simulink model "TrajectoryTracking_2015b_00"  (R2017a)
settings: Solver=ode45  StartTime=0.0  StopTime=200  RelTol=1e-3
values from neighbouring files (symbols this model uses):
  B_input = B_T    [ErrorDynamicsControllerDesign.m]
  tau_d_1 = C_RB1+C_A1+D1+G1    [DesiredInputOptimalConfiguration.m]
  tau_d_2 = C_RB2+C_A2+D2+G2    [DesiredInputOptimalConfiguration.m]
  tau_d_3 = C_RB3+C_A3+D3+G3    [DesiredInputOptimalConfiguration.m]
  tau_d_4 = C_RB4+C_A4+D4+G4    [DesiredInputOptimalConfiguration.m]
  tau_d_5 = C_RB5+C_A5+D5+G5    [DesiredInputOptimalConfiguration.m]
  tau_d_6 = C_RB6+C_A6+D6+G6    [DesiredInputOptimalConfiguration.m]
  tau_d_7 = C_RB7+C_A7+D7+G7    [DesiredInputOptimalConfiguration.m]
undefined symbols (not defined in the file or in its folder): angular_velocity_pitch_1, angular_velocity_pitch_2, angular_velocity_pitch_3, angular_velocity_pitch_4, angular_velocity_pitch_5, angular_velocity_pitch_6, angular_velocity_roll_1, angular_velocity_roll_2, angular_velocity_roll_3, angular_velocity_roll_4, angular_velocity_roll_5, angular_velocity_roll_6, angular_velocity_roll_7, angular_velocity_yaw_1, angular_velocity_yaw_2, angular_velocity_yaw_3, angular_velocity_yaw_4, angular_velocity_yaw_5, angular_velocity_yaw_6, angular_velocity_yaw_7, K1, K2, K3, K4, K5, K6, K7, linear_velocity_x_1, linear_velocity_x_2, linear_velocity_x_3, linear_velocity_x_4, linear_velocity_x_5, linear_velocity_x_6, linear_velocity_x_7, linear_velocity_y_1, linear_velocity_y_2, linear_velocity_y_3, linear_velocity_y_4, linear_velocity_y_5, linear_velocity_y_6, linear_velocity_y_7, linear_velocity_z_1, linear_velocity_z_2, linear_velocity_z_3, linear_velocity_z_4, linear_velocity_z_5, linear_velocity_z_6, linear_velocity_z_7, pitch_angle_1, pitch_angle_2, pitch_angle_3, pitch_angle_4, pitch_angle_5, pitch_angle_6, pitch_angle_7, roll_angle_1, roll_angle_2, roll_angle_3, roll_angle_4, roll_angle_5 ... (+52)
undefined symbols (not defined in the file): b_T1_optimized, b_T2_optimized, b_T3_optimized, b_T4_optimized, b_T5_optimized, b_T6_optimized, d_T1_optimized, d_T2_optimized, d_T3_optimized, d_T4_optimized, d_T5_optimized, d_T6_optimized, r_T1_optimized, r_T2_optimized, r_T3_optimized, r_T4_optimized, r_T5_optimized, r_T6_optimized
libraries: sharedtransform x1, shared6dofsys x1
(part 2 of 2)

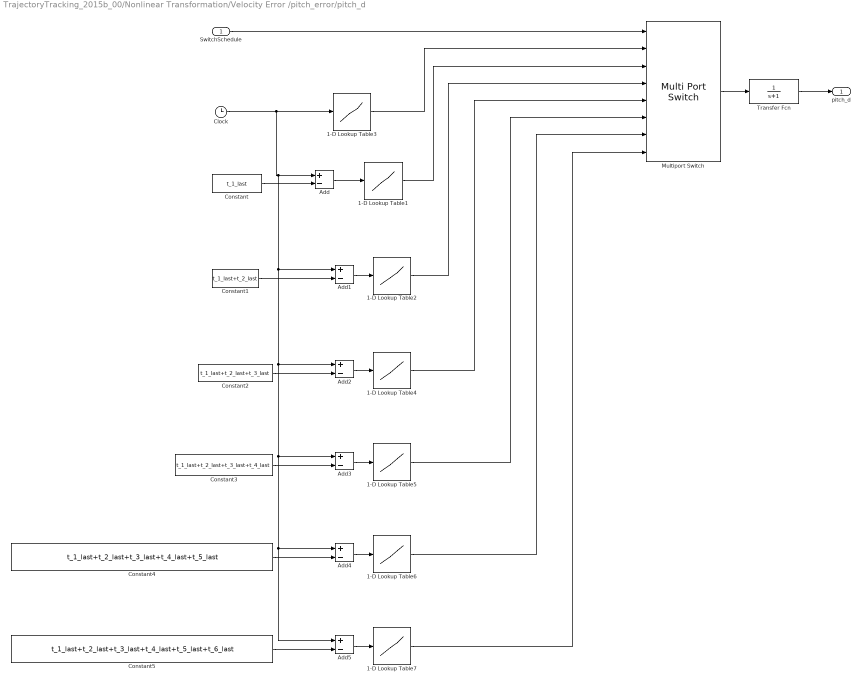
== system TrajectoryTracking_2015b_00/Nonlinear Transformation/Velocity Error /pitch_error/pitch_d ==
  SwitchSchedule : Inport
  1-D Lookup Table1 : Lookup_n-D  NumberOfTableDimensions=1  BreakpointsForDimension1=t_e_2  Table=angular_velocity_pitch_2  InternalRulePriority=Speed  RndMeth=Simplest  InputSameDT=on
  1-D Lookup Table2 : Lookup_n-D  NumberOfTableDimensions=1  BreakpointsForDimension1=t_e_3  Table=angular_velocity_pitch_3  InternalRulePriority=Speed  RndMeth=Simplest  InputSameDT=on
  1-D Lookup Table3 : Lookup_n-D  NumberOfTableDimensions=1  BreakpointsForDimension1=t_e_1  Table=angular_velocity_pitch_1  InternalRulePriority=Speed  RndMeth=Simplest  InputSameDT=on
  1-D Lookup Table4 : Lookup_n-D  NumberOfTableDimensions=1  BreakpointsForDimension1=t_e_4  Table=angular_velocity_pitch_4  InternalRulePriority=Speed  RndMeth=Simplest  InputSameDT=on
  1-D Lookup Table5 : Lookup_n-D  NumberOfTableDimensions=1  BreakpointsForDimension1=t_e_5  Table=angular_velocity_pitch_5  InternalRulePriority=Speed  RndMeth=Simplest  InputSameDT=on
  1-D Lookup Table6 : Lookup_n-D  NumberOfTableDimensions=1  BreakpointsForDimension1=t_e_6  Table=angular_velocity_pitch_6  InternalRulePriority=Speed  RndMeth=Simplest  InputSameDT=on
  1-D Lookup Table7 : Lookup_n-D  NumberOfTableDimensions=1  BreakpointsForDimension1=t_e_6  Table=angular_velocity_pitch_6  InternalRulePriority=Speed  RndMeth=Simplest  InputSameDT=on
  Add{,1..5} (6 alike) : Sum  Inputs=+-
  Clock : Clock
  Constant : Constant  Value=t_1_last
  Constant1 : Constant  Value=t_1_last+t_2_last
  Constant2 : Constant  Value=t_1_last+t_2_last+t_3_last
  Constant3 : Constant  Value=t_1_last+t_2_last+t_3_last+t_4_last
  Constant4 : Constant  Value=t_1_last+t_2_last+t_3_last+t_4_last+t_5_last
  Constant5 : Constant  Value=t_1_last+t_2_last+t_3_last+t_4_last+t_5_last+t_6_last
  Multiport Switch : MultiPortSwitch  Inputs=7
  Transfer Fcn : TransferFcn  Denominator=[1 1]
  pitch_d : Outport
  wires:
  1-D Lookup Table1/1 -> Multiport Switch/3
  1-D Lookup Table3/1 -> Multiport Switch/2
  Constant/1 -> Add/2
  Multiport Switch/1 -> Transfer Fcn/1
  SwitchSchedule/1 -> Multiport Switch/1
  Clock/1 -> Add5/1, Add4/1, Add3/1, Add2/1, Add1/1, Add/1, 1-D Lookup Table3/1
  Add/1 -> 1-D Lookup Table1/1
  1-D Lookup Table2/1 -> Multiport Switch/4
  Constant1/1 -> Add1/2
  Add1/1 -> 1-D Lookup Table2/1
  Constant2/1 -> Add2/2
  Add2/1 -> 1-D Lookup Table4/1
  1-D Lookup Table4/1 -> Multiport Switch/5
  Transfer Fcn/1 -> pitch_d/1
  Constant3/1 -> Add3/2
  Add3/1 -> 1-D Lookup Table5/1
  1-D Lookup Table5/1 -> Multiport Switch/6
  Add4/1 -> 1-D Lookup Table6/1
  Constant4/1 -> Add4/2
  1-D Lookup Table6/1 -> Multiport Switch/7
  Add5/1 -> 1-D Lookup Table7/1
  Constant5/1 -> Add5/2
  1-D Lookup Table7/1 -> Multiport Switch/8

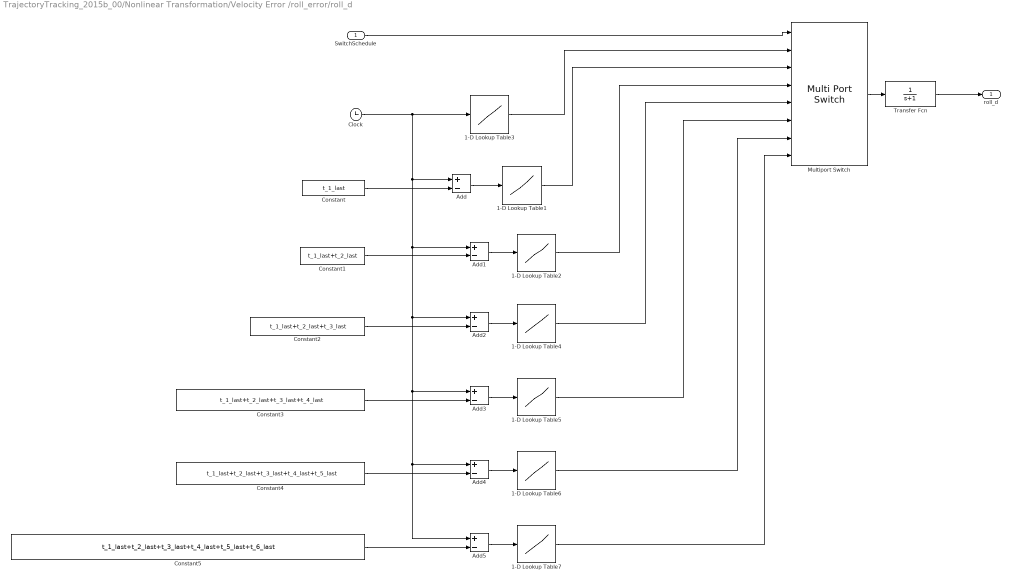
== system TrajectoryTracking_2015b_00/Nonlinear Transformation/Velocity Error /roll_error/roll_d ==
  SwitchSchedule : Inport
  1-D Lookup Table1 : Lookup_n-D  NumberOfTableDimensions=1  BreakpointsForDimension1=t_e_2  Table=angular_velocity_roll_2  InternalRulePriority=Speed  RndMeth=Simplest  InputSameDT=on
  1-D Lookup Table2 : Lookup_n-D  NumberOfTableDimensions=1  BreakpointsForDimension1=t_e_3  Table=angular_velocity_roll_3  InternalRulePriority=Speed  RndMeth=Simplest  InputSameDT=on
  1-D Lookup Table3 : Lookup_n-D  NumberOfTableDimensions=1  BreakpointsForDimension1=t_e_1  Table=angular_velocity_roll_1  InternalRulePriority=Speed  RndMeth=Simplest  InputSameDT=on
  1-D Lookup Table4 : Lookup_n-D  NumberOfTableDimensions=1  BreakpointsForDimension1=t_e_4  Table=angular_velocity_roll_4  InternalRulePriority=Speed  RndMeth=Simplest  InputSameDT=on
  1-D Lookup Table5 : Lookup_n-D  NumberOfTableDimensions=1  BreakpointsForDimension1=t_e_5  Table=angular_velocity_roll_5  InternalRulePriority=Speed  RndMeth=Simplest  InputSameDT=on
  1-D Lookup Table6 : Lookup_n-D  NumberOfTableDimensions=1  BreakpointsForDimension1=t_e_6  Table=angular_velocity_roll_6  InternalRulePriority=Speed  RndMeth=Simplest  InputSameDT=on
  1-D Lookup Table7 : Lookup_n-D  NumberOfTableDimensions=1  BreakpointsForDimension1=t_e_7  Table=angular_velocity_roll_7  InternalRulePriority=Speed  RndMeth=Simplest  InputSameDT=on
  Add{,1..5} (6 alike) : Sum  Inputs=+-
  Clock : Clock
  Constant : Constant  Value=t_1_last
  Constant1 : Constant  Value=t_1_last+t_2_last
  Constant2 : Constant  Value=t_1_last+t_2_last+t_3_last
  Constant3 : Constant  Value=t_1_last+t_2_last+t_3_last+t_4_last
  Constant4 : Constant  Value=t_1_last+t_2_last+t_3_last+t_4_last+t_5_last
  Constant5 : Constant  Value=t_1_last+t_2_last+t_3_last+t_4_last+t_5_last+t_6_last
  Multiport Switch : MultiPortSwitch  Inputs=7
  Transfer Fcn : TransferFcn  Denominator=[1 1]
  roll_d : Outport
  wires:
  1-D Lookup Table1/1 -> Multiport Switch/3
  1-D Lookup Table3/1 -> Multiport Switch/2
  Constant/1 -> Add/2
  Multiport Switch/1 -> Transfer Fcn/1
  SwitchSchedule/1 -> Multiport Switch/1
  Clock/1 -> Add5/1, Add4/1, Add3/1, Add2/1, Add1/1, Add/1, 1-D Lookup Table3/1
  Add/1 -> 1-D Lookup Table1/1
  Constant1/1 -> Add1/2
  Add1/1 -> 1-D Lookup Table2/1
  1-D Lookup Table2/1 -> Multiport Switch/4
  Add2/1 -> 1-D Lookup Table4/1
  Constant2/1 -> Add2/2
  1-D Lookup Table4/1 -> Multiport Switch/5
  Transfer Fcn/1 -> roll_d/1
  Constant3/1 -> Add3/2
  Add3/1 -> 1-D Lookup Table5/1
  1-D Lookup Table5/1 -> Multiport Switch/6
  Constant4/1 -> Add4/2
  Add4/1 -> 1-D Lookup Table6/1
  1-D Lookup Table6/1 -> Multiport Switch/7
  Add5/1 -> 1-D Lookup Table7/1
  Constant5/1 -> Add5/2
  1-D Lookup Table7/1 -> Multiport Switch/8

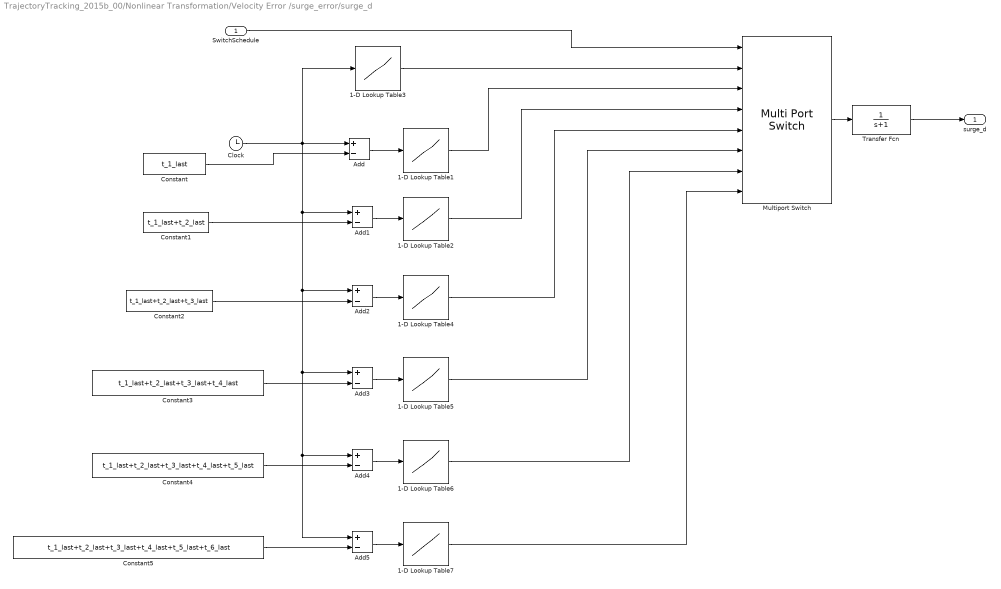
== system TrajectoryTracking_2015b_00/Nonlinear Transformation/Velocity Error /surge_error/surge_d ==
  SwitchSchedule : Inport
  1-D Lookup Table1 : Lookup_n-D  NumberOfTableDimensions=1  BreakpointsForDimension1=t_e_2  Table=linear_velocity_x_2  InternalRulePriority=Speed  RndMeth=Simplest  InputSameDT=on
  1-D Lookup Table2 : Lookup_n-D  NumberOfTableDimensions=1  BreakpointsForDimension1=t_e_3  Table=linear_velocity_x_3  InternalRulePriority=Speed  RndMeth=Simplest  InputSameDT=on
  1-D Lookup Table3 : Lookup_n-D  NumberOfTableDimensions=1  BreakpointsForDimension1=t_e_1  Table=linear_velocity_x_1  InternalRulePriority=Speed  RndMeth=Simplest  InputSameDT=on
  1-D Lookup Table4 : Lookup_n-D  NumberOfTableDimensions=1  BreakpointsForDimension1=t_e_4  Table=linear_velocity_x_4  InternalRulePriority=Speed  RndMeth=Simplest  InputSameDT=on
  1-D Lookup Table5 : Lookup_n-D  NumberOfTableDimensions=1  BreakpointsForDimension1=t_e_5  Table=linear_velocity_x_5  InternalRulePriority=Speed  RndMeth=Simplest  InputSameDT=on
  1-D Lookup Table6 : Lookup_n-D  NumberOfTableDimensions=1  BreakpointsForDimension1=t_e_6  Table=linear_velocity_x_6  InternalRulePriority=Speed  RndMeth=Simplest  InputSameDT=on
  1-D Lookup Table7 : Lookup_n-D  NumberOfTableDimensions=1  BreakpointsForDimension1=t_e_7  Table=linear_velocity_x_7  InternalRulePriority=Speed  RndMeth=Simplest  InputSameDT=on
  Add{,1..5} (6 alike) : Sum  Inputs=+-
  Clock : Clock
  Constant : Constant  Value=t_1_last
  Constant1 : Constant  Value=t_1_last+t_2_last
  Constant2 : Constant  Value=t_1_last+t_2_last+t_3_last
  Constant3 : Constant  Value=t_1_last+t_2_last+t_3_last+t_4_last
  Constant4 : Constant  Value=t_1_last+t_2_last+t_3_last+t_4_last+t_5_last
  Constant5 : Constant  Value=t_1_last+t_2_last+t_3_last+t_4_last+t_5_last+t_6_last
  Multiport Switch : MultiPortSwitch  Inputs=7
  Transfer Fcn : TransferFcn  Denominator=[1 1]
  surge_d : Outport
  wires:
  1-D Lookup Table1/1 -> Multiport Switch/3
  1-D Lookup Table3/1 -> Multiport Switch/2
  Constant/1 -> Add/2
  Multiport Switch/1 -> Transfer Fcn/1
  SwitchSchedule/1 -> Multiport Switch/1
  Clock/1 -> Add5/1, Add4/1, Add3/1, Add2/1, Add1/1, Add/1, 1-D Lookup Table3/1
  Add/1 -> 1-D Lookup Table1/1
  Constant1/1 -> Add1/2
  Add1/1 -> 1-D Lookup Table2/1
  1-D Lookup Table2/1 -> Multiport Switch/4
  Constant2/1 -> Add2/2
  Add2/1 -> 1-D Lookup Table4/1
  1-D Lookup Table4/1 -> Multiport Switch/5
  Transfer Fcn/1 -> surge_d/1
  Add3/1 -> 1-D Lookup Table5/1
  Constant3/1 -> Add3/2
  1-D Lookup Table5/1 -> Multiport Switch/6
  Constant4/1 -> Add4/2
  Add4/1 -> 1-D Lookup Table6/1
  1-D Lookup Table6/1 -> Multiport Switch/7
  Constant5/1 -> Add5/2
  Add5/1 -> 1-D Lookup Table7/1
  1-D Lookup Table7/1 -> Multiport Switch/8

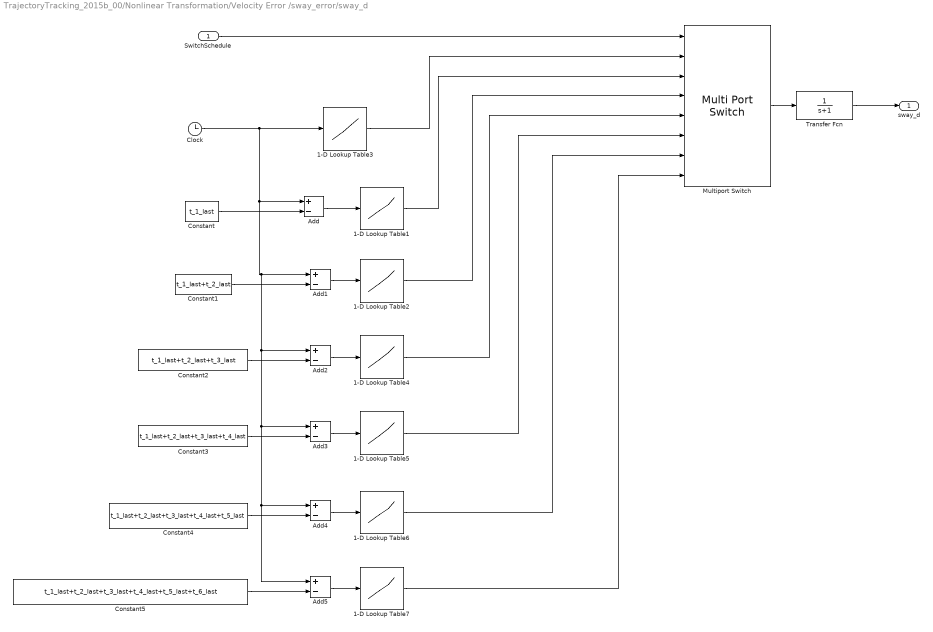
== system TrajectoryTracking_2015b_00/Nonlinear Transformation/Velocity Error /sway_error/sway_d ==
  SwitchSchedule : Inport
  1-D Lookup Table1 : Lookup_n-D  NumberOfTableDimensions=1  BreakpointsForDimension1=t_e_2  Table=linear_velocity_y_2  InternalRulePriority=Speed  RndMeth=Simplest  InputSameDT=on
  1-D Lookup Table2 : Lookup_n-D  NumberOfTableDimensions=1  BreakpointsForDimension1=t_e_3  Table=linear_velocity_y_3  InternalRulePriority=Speed  RndMeth=Simplest  InputSameDT=on
  1-D Lookup Table3 : Lookup_n-D  NumberOfTableDimensions=1  BreakpointsForDimension1=t_e_1  Table=linear_velocity_y_1  InternalRulePriority=Speed  RndMeth=Simplest  InputSameDT=on
  1-D Lookup Table4 : Lookup_n-D  NumberOfTableDimensions=1  BreakpointsForDimension1=t_e_4  Table=linear_velocity_y_4  InternalRulePriority=Speed  RndMeth=Simplest  InputSameDT=on
  1-D Lookup Table5 : Lookup_n-D  NumberOfTableDimensions=1  BreakpointsForDimension1=t_e_5  Table=linear_velocity_y_5  InternalRulePriority=Speed  RndMeth=Simplest  InputSameDT=on
  1-D Lookup Table6 : Lookup_n-D  NumberOfTableDimensions=1  BreakpointsForDimension1=t_e_6  Table=linear_velocity_y_6  InternalRulePriority=Speed  RndMeth=Simplest  InputSameDT=on
  1-D Lookup Table7 : Lookup_n-D  NumberOfTableDimensions=1  BreakpointsForDimension1=t_e_7  Table=linear_velocity_y_7  InternalRulePriority=Speed  RndMeth=Simplest  InputSameDT=on
  Add{,1..5} (6 alike) : Sum  Inputs=+-
  Clock : Clock
  Constant : Constant  Value=t_1_last
  Constant1 : Constant  Value=t_1_last+t_2_last
  Constant2 : Constant  Value=t_1_last+t_2_last+t_3_last
  Constant3 : Constant  Value=t_1_last+t_2_last+t_3_last+t_4_last
  Constant4 : Constant  Value=t_1_last+t_2_last+t_3_last+t_4_last+t_5_last
  Constant5 : Constant  Value=t_1_last+t_2_last+t_3_last+t_4_last+t_5_last+t_6_last
  Multiport Switch : MultiPortSwitch  Inputs=7
  Transfer Fcn : TransferFcn  Denominator=[1 1]
  sway_d : Outport
  wires:
  1-D Lookup Table1/1 -> Multiport Switch/3
  1-D Lookup Table3/1 -> Multiport Switch/2
  Constant/1 -> Add/2
  Multiport Switch/1 -> Transfer Fcn/1
  SwitchSchedule/1 -> Multiport Switch/1
  Clock/1 -> Add/1, Add5/1, Add4/1, Add3/1, Add2/1, Add1/1, 1-D Lookup Table3/1
  Add/1 -> 1-D Lookup Table1/1
  Constant1/1 -> Add1/2
  Add1/1 -> 1-D Lookup Table2/1
  1-D Lookup Table2/1 -> Multiport Switch/4
  Constant2/1 -> Add2/2
  Add2/1 -> 1-D Lookup Table4/1
  1-D Lookup Table4/1 -> Multiport Switch/5
  Transfer Fcn/1 -> sway_d/1
  Add3/1 -> 1-D Lookup Table5/1
  Constant3/1 -> Add3/2
  1-D Lookup Table5/1 -> Multiport Switch/6
  Constant4/1 -> Add4/2
  Add4/1 -> 1-D Lookup Table6/1
  1-D Lookup Table6/1 -> Multiport Switch/7
  Constant5/1 -> Add5/2
  Add5/1 -> 1-D Lookup Table7/1
  1-D Lookup Table7/1 -> Multiport Switch/8

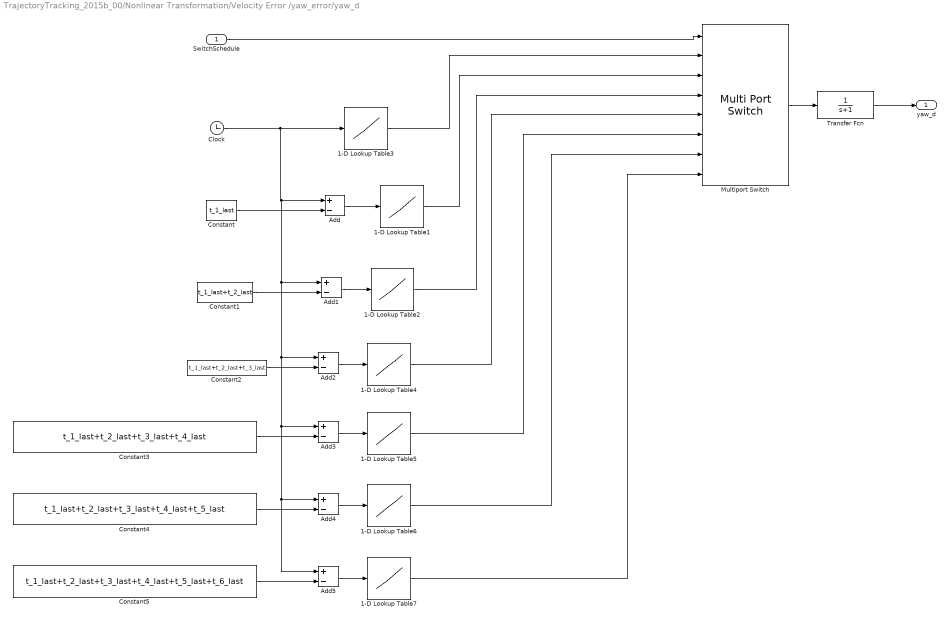
== system TrajectoryTracking_2015b_00/Nonlinear Transformation/Velocity Error /yaw_error/yaw_d ==
  SwitchSchedule : Inport
  1-D Lookup Table1 : Lookup_n-D  NumberOfTableDimensions=1  BreakpointsForDimension1=t_e_2  Table=angular_velocity_yaw_2  InternalRulePriority=Speed  RndMeth=Simplest  InputSameDT=on
  1-D Lookup Table2 : Lookup_n-D  NumberOfTableDimensions=1  BreakpointsForDimension1=t_e_3  Table=angular_velocity_yaw_3  InternalRulePriority=Speed  RndMeth=Simplest  InputSameDT=on
  1-D Lookup Table3 : Lookup_n-D  NumberOfTableDimensions=1  BreakpointsForDimension1=t_e_1  Table=angular_velocity_yaw_1  InternalRulePriority=Speed  RndMeth=Simplest  InputSameDT=on
  1-D Lookup Table4 : Lookup_n-D  NumberOfTableDimensions=1  BreakpointsForDimension1=t_e_4  Table=angular_velocity_yaw_4  InternalRulePriority=Speed  RndMeth=Simplest  InputSameDT=on
  1-D Lookup Table5 : Lookup_n-D  NumberOfTableDimensions=1  BreakpointsForDimension1=t_e_5  Table=angular_velocity_yaw_5  InternalRulePriority=Speed  RndMeth=Simplest  InputSameDT=on
  1-D Lookup Table6 : Lookup_n-D  NumberOfTableDimensions=1  BreakpointsForDimension1=t_e_6  Table=angular_velocity_yaw_6  InternalRulePriority=Speed  RndMeth=Simplest  InputSameDT=on
  1-D Lookup Table7 : Lookup_n-D  NumberOfTableDimensions=1  BreakpointsForDimension1=t_e_7  Table=angular_velocity_yaw_7  InternalRulePriority=Speed  RndMeth=Simplest  InputSameDT=on
  Add{,1..5} (6 alike) : Sum  Inputs=+-
  Clock : Clock
  Constant : Constant  Value=t_1_last
  Constant1 : Constant  Value=t_1_last+t_2_last
  Constant2 : Constant  Value=t_1_last+t_2_last+t_3_last
  Constant3 : Constant  Value=t_1_last+t_2_last+t_3_last+t_4_last
  Constant4 : Constant  Value=t_1_last+t_2_last+t_3_last+t_4_last+t_5_last
  Constant5 : Constant  Value=t_1_last+t_2_last+t_3_last+t_4_last+t_5_last+t_6_last
  Multiport Switch : MultiPortSwitch  Inputs=7
  Transfer Fcn : TransferFcn  Denominator=[1 1]
  yaw_d : Outport
  wires:
  1-D Lookup Table1/1 -> Multiport Switch/3
  1-D Lookup Table3/1 -> Multiport Switch/2
  Constant/1 -> Add/2
  Multiport Switch/1 -> Transfer Fcn/1
  SwitchSchedule/1 -> Multiport Switch/1
  Clock/1 -> Add5/1, Add4/1, Add3/1, Add2/1, Add1/1, Add/1, 1-D Lookup Table3/1
  Add/1 -> 1-D Lookup Table1/1
  1-D Lookup Table2/1 -> Multiport Switch/4
  Constant1/1 -> Add1/2
  Add1/1 -> 1-D Lookup Table2/1
  Constant2/1 -> Add2/2
  Add2/1 -> 1-D Lookup Table4/1
  Transfer Fcn/1 -> yaw_d/1
  Add3/1 -> 1-D Lookup Table5/1
  Constant3/1 -> Add3/2
  1-D Lookup Table4/1 -> Multiport Switch/5
  1-D Lookup Table5/1 -> Multiport Switch/6
  Add4/1 -> 1-D Lookup Table6/1
  Constant4/1 -> Add4/2
  1-D Lookup Table6/1 -> Multiport Switch/7
  Constant5/1 -> Add5/2
  Add5/1 -> 1-D Lookup Table7/1
  1-D Lookup Table7/1 -> Multiport Switch/8

== system TrajectoryTracking_2015b_00/Underwater Robot System/Underwater Robot System/Dynamic2Kinematic(angular velocity)/Initial Integration Phi ==
  Constant : Constant  Value=0
  Initial Phi Integration Value : Outport
  wires:
  Constant/1 -> Initial Phi Integration Value/1

== system TrajectoryTracking_2015b_00/Underwater Robot System/Underwater Robot System/Dynamic2Kinematic(angular velocity)/Initial Integration Value Generation Psi ==
  Constant : Constant  Value=0
  Initial Orientation Integration Value : Outport
  wires:
  Constant/1 -> Initial Orientation Integration Value/1

== system TrajectoryTracking_2015b_00/Underwater Robot System/Underwater Robot System/Dynamic2Kinematic(angular velocity)/Initial Integration Value Generation Theta ==
  Constant : Constant  Value=0
  Initial Theta Integration Value : Outport
  wires:
  Constant/1 -> Initial Theta Integration Value/1

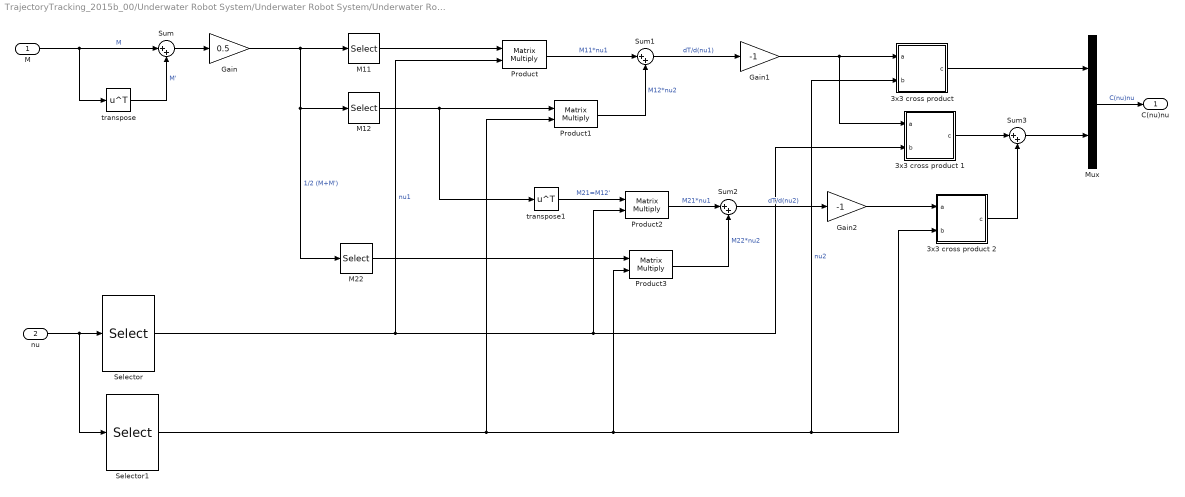
== system TrajectoryTracking_2015b_00/Underwater Robot System/Underwater Robot System/Underwater Robot Dynamics /6DOF Coriolis forces ==
  M : Inport
  nu : Inport  Port=2
  3x3 cross product : Subsystem
  3x3 cross product 1 : Subsystem
  3x3 cross product 2 : Subsystem
  Gain : Gain  Gain=0.5  SaturateOnIntegerOverflow=on  OutDataTypeStr=Inherit: Same as input  ParamDataTypeStr=Inherit: Same as input
  Gain1 : Gain  Gain=-1  SaturateOnIntegerOverflow=on  OutDataTypeStr=Inherit: Same as input  ParamDataTypeStr=Inherit: Same as input
  Gain2 : Gain  Gain=-1  SaturateOnIntegerOverflow=on  OutDataTypeStr=Inherit: Same as input  ParamDataTypeStr=Inherit: Same as input
  M11 : Selector  NumberOfDimensions=2  InputPortWidth=3  IndexOptions=Index vector (dialog),Index vector (dialog)  Indices=[1 2 3],[1 2 3]  OutputSizes=1
  M12 : Selector  NumberOfDimensions=2  InputPortWidth=3  IndexOptions=Index vector (dialog),Index vector (dialog)  Indices=[1 2 3],[4 5 6]  OutputSizes=1
  M22 : Selector  NumberOfDimensions=2  InputPortWidth=3  IndexOptions=Index vector (dialog),Index vector (dialog)  Indices=[4 5 6],[4 5 6]  OutputSizes=1
  Mux : Mux  Inputs=2
  Product{,1..3} (4 alike) : Product  Multiplication=Matrix(*)  SaturateOnIntegerOverflow=on  OutDataTypeStr=Inherit: Same as first input
  Selector : Selector  InputPortWidth=6  IndexOptions=Index vector (dialog)  Indices=[1 2 3]  OutputSizes=1
  Selector1 : Selector  InputPortWidth=6  IndexOptions=Index vector (dialog)  Indices=[4 5 6]  OutputSizes=1
  Sum{,1..3} (4 alike) : Sum  Inputs=|++  SaturateOnIntegerOverflow=on
  transpose : Math  Operator=transpose  SaturateOnIntegerOverflow=on
  transpose1 : Math  Operator=transpose  SaturateOnIntegerOverflow=on
  C(nu)nu : Outport
  wires:
  transpose/1 -> Sum/2  "M'"
  Sum/1 -> Gain/1
  Gain/1 -> M22/1, M12/1, M11/1  "1/2 (M+M')"
  Selector/1 -> Product2/2, 3x3 cross product 1/2(b), Product/2  "nu1"
  Selector1/1 -> 3x3 cross product/2(b), 3x3 cross product 2/2(b), Product3/2, Product1/2  "nu2"
  M11/1 -> Product/1
  Product/1 -> Sum1/1  "M11*nu1"
  M12/1 -> transpose1/1, Product1/1
  Product1/1 -> Sum1/2  "M12*nu2"
  Sum1/1 -> Gain1/1  "dT/d(nu1)"
  transpose1/1 -> Product2/1  "M21=M12'"
  Product2/1 -> Sum2/1  "M21*nu1"
  M22/1 -> Product3/1
  Product3/1 -> Sum2/2  "M22*nu2"
  Sum2/1 -> Gain2/1  "dT/d(nu2)"
  Gain1/1 -> 3x3 cross product/1(a), 3x3 cross product 1/1(a)
  3x3 cross product/1(c) -> Mux/1
  Gain2/1 -> 3x3 cross product 2/1(a)
  3x3 cross product 1/1(c) -> Sum3/1
  3x3 cross product 2/1(c) -> Sum3/2
  Sum3/1 -> Mux/2
  Mux/1 -> C(nu)nu/1  "C(nu)nu"
  nu/1 -> Selector/1, Selector1/1
  M/1 -> transpose/1, Sum/1  "M"

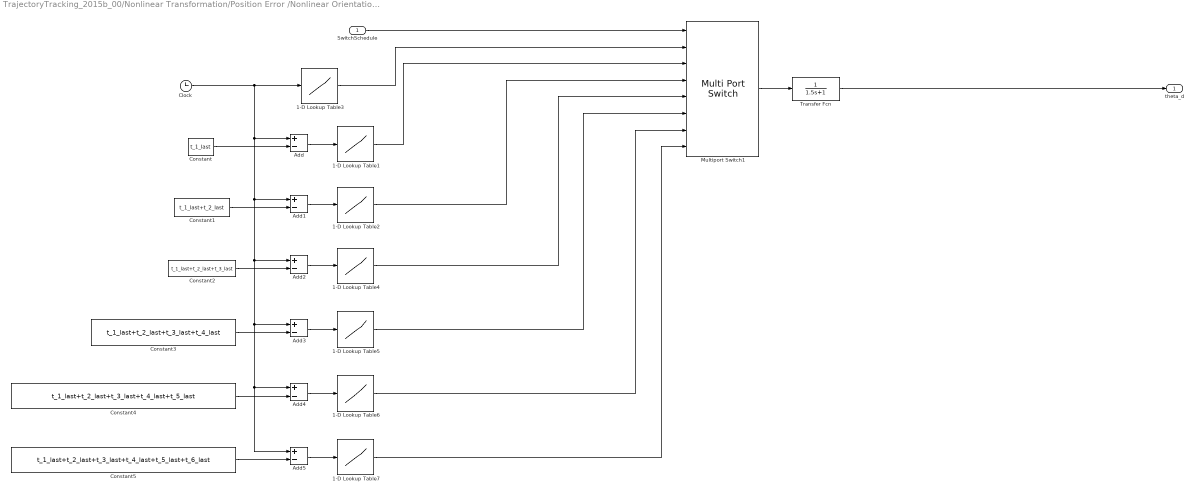
== system TrajectoryTracking_2015b_00/Nonlinear Transformation/Position Error /Nonlinear Orientation Transformation/pitch_error/theta_d ==
  SwitchSchedule : Inport
  1-D Lookup Table1 : Lookup_n-D  NumberOfTableDimensions=1  BreakpointsForDimension1=t_e_2  Table=pitch_angle_2  InternalRulePriority=Speed  RndMeth=Simplest  InputSameDT=on
  1-D Lookup Table2 : Lookup_n-D  NumberOfTableDimensions=1  BreakpointsForDimension1=t_e_3  Table=pitch_angle_3  InternalRulePriority=Speed  RndMeth=Simplest  InputSameDT=on
  1-D Lookup Table3 : Lookup_n-D  NumberOfTableDimensions=1  BreakpointsForDimension1=t_e_1  Table=pitch_angle_1  InternalRulePriority=Speed  RndMeth=Simplest  InputSameDT=on
  1-D Lookup Table4 : Lookup_n-D  NumberOfTableDimensions=1  BreakpointsForDimension1=t_e_4  Table=pitch_angle_4  InternalRulePriority=Speed  RndMeth=Simplest  InputSameDT=on
  1-D Lookup Table5 : Lookup_n-D  NumberOfTableDimensions=1  BreakpointsForDimension1=t_e_5  Table=pitch_angle_5  InternalRulePriority=Speed  RndMeth=Simplest  InputSameDT=on
  1-D Lookup Table6 : Lookup_n-D  NumberOfTableDimensions=1  BreakpointsForDimension1=t_e_6  Table=pitch_angle_6  InternalRulePriority=Speed  RndMeth=Simplest  InputSameDT=on
  1-D Lookup Table7 : Lookup_n-D  NumberOfTableDimensions=1  BreakpointsForDimension1=t_e_7  Table=pitch_angle_7  InternalRulePriority=Speed  RndMeth=Simplest  InputSameDT=on
  Add{,1..5} (6 alike) : Sum  Inputs=+-
  Clock : Clock
  Constant : Constant  Value=t_1_last
  Constant1 : Constant  Value=t_1_last+t_2_last
  Constant2 : Constant  Value=t_1_last+t_2_last+t_3_last
  Constant3 : Constant  Value=t_1_last+t_2_last+t_3_last+t_4_last
  Constant4 : Constant  Value=t_1_last+t_2_last+t_3_last+t_4_last+t_5_last
  Constant5 : Constant  Value=t_1_last+t_2_last+t_3_last+t_4_last+t_5_last+t_6_last
  Multiport Switch1 : MultiPortSwitch  Inputs=7
  Transfer Fcn : TransferFcn  Denominator=[1.5 1]
  theta_d : Outport
  wires:
  SwitchSchedule/1 -> Multiport Switch1/1
  1-D Lookup Table1/1 -> Multiport Switch1/3
  1-D Lookup Table3/1 -> Multiport Switch1/2
  Constant/1 -> Add/2
  Multiport Switch1/1 -> Transfer Fcn/1
  Clock/1 -> Add5/1, Add4/1, Add3/1, Add2/1, Add1/1, Add/1, 1-D Lookup Table3/1
  Add/1 -> 1-D Lookup Table1/1
  Add1/1 -> 1-D Lookup Table2/1
  1-D Lookup Table2/1 -> Multiport Switch1/4
  Constant1/1 -> Add1/2
  Constant2/1 -> Add2/2
  Add2/1 -> 1-D Lookup Table4/1
  1-D Lookup Table4/1 -> Multiport Switch1/5
  Constant3/1 -> Add3/2
  Add3/1 -> 1-D Lookup Table5/1
  1-D Lookup Table5/1 -> Multiport Switch1/6
  Add4/1 -> 1-D Lookup Table6/1
  Constant4/1 -> Add4/2
  1-D Lookup Table6/1 -> Multiport Switch1/7
  Constant5/1 -> Add5/2
  Add5/1 -> 1-D Lookup Table7/1
  1-D Lookup Table7/1 -> Multiport Switch1/8
  Transfer Fcn/1 -> theta_d/1

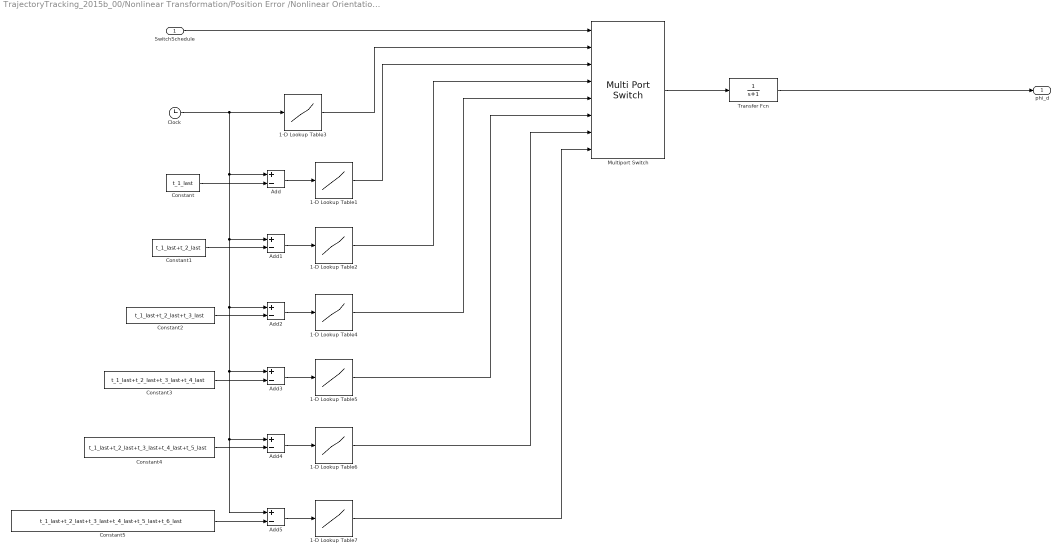
== system TrajectoryTracking_2015b_00/Nonlinear Transformation/Position Error /Nonlinear Orientation Transformation/roll_error/phi_d ==
  SwitchSchedule : Inport
  1-D Lookup Table1 : Lookup_n-D  NumberOfTableDimensions=1  BreakpointsForDimension1=t_e_2  Table=roll_angle_2  InternalRulePriority=Speed  RndMeth=Simplest  InputSameDT=on
  1-D Lookup Table2 : Lookup_n-D  NumberOfTableDimensions=1  BreakpointsForDimension1=t_e_3  Table=roll_angle_3  InternalRulePriority=Speed  RndMeth=Simplest  InputSameDT=on
  1-D Lookup Table3 : Lookup_n-D  NumberOfTableDimensions=1  BreakpointsForDimension1=t_e_1  Table=roll_angle_1  InternalRulePriority=Speed  RndMeth=Simplest  InputSameDT=on
  1-D Lookup Table4 : Lookup_n-D  NumberOfTableDimensions=1  BreakpointsForDimension1=t_e_4  Table=roll_angle_4  InternalRulePriority=Speed  RndMeth=Simplest  InputSameDT=on
  1-D Lookup Table5 : Lookup_n-D  NumberOfTableDimensions=1  BreakpointsForDimension1=t_e_5  Table=roll_angle_5  InternalRulePriority=Speed  RndMeth=Simplest  InputSameDT=on
  1-D Lookup Table6 : Lookup_n-D  NumberOfTableDimensions=1  BreakpointsForDimension1=t_e_6  Table=roll_angle_6  InternalRulePriority=Speed  RndMeth=Simplest  InputSameDT=on
  1-D Lookup Table7 : Lookup_n-D  NumberOfTableDimensions=1  BreakpointsForDimension1=t_e_7  Table=roll_angle_7  InternalRulePriority=Speed  RndMeth=Simplest  InputSameDT=on
  Add{,1..5} (6 alike) : Sum  Inputs=+-
  Clock : Clock
  Constant : Constant  Value=t_1_last
  Constant1 : Constant  Value=t_1_last+t_2_last
  Constant2 : Constant  Value=t_1_last+t_2_last+t_3_last
  Constant3 : Constant  Value=t_1_last+t_2_last+t_3_last+t_4_last
  Constant4 : Constant  Value=t_1_last+t_2_last+t_3_last+t_4_last+t_5_last
  Constant5 : Constant  Value=t_1_last+t_2_last+t_3_last+t_4_last+t_5_last+t_6_last
  Multiport Switch : MultiPortSwitch  Inputs=7
  Transfer Fcn : TransferFcn  Denominator=[1 1]
  phi_d : Outport
  wires:
  1-D Lookup Table1/1 -> Multiport Switch/3
  1-D Lookup Table3/1 -> Multiport Switch/2
  Constant/1 -> Add/2
  Multiport Switch/1 -> Transfer Fcn/1
  Clock/1 -> Add1/1, Add5/1, Add4/1, Add3/1, Add2/1, Add/1, 1-D Lookup Table3/1
  Add/1 -> 1-D Lookup Table1/1
  SwitchSchedule/1 -> Multiport Switch/1
  Constant1/1 -> Add1/2
  Add1/1 -> 1-D Lookup Table2/1
  1-D Lookup Table2/1 -> Multiport Switch/4
  Add2/1 -> 1-D Lookup Table4/1
  Constant2/1 -> Add2/2
  1-D Lookup Table4/1 -> Multiport Switch/5
  Constant3/1 -> Add3/2
  Add3/1 -> 1-D Lookup Table5/1
  1-D Lookup Table5/1 -> Multiport Switch/6
  Add4/1 -> 1-D Lookup Table6/1
  Constant4/1 -> Add4/2
  1-D Lookup Table6/1 -> Multiport Switch/7
  Add5/1 -> 1-D Lookup Table7/1
  Constant5/1 -> Add5/2
  1-D Lookup Table7/1 -> Multiport Switch/8
  Transfer Fcn/1 -> phi_d/1

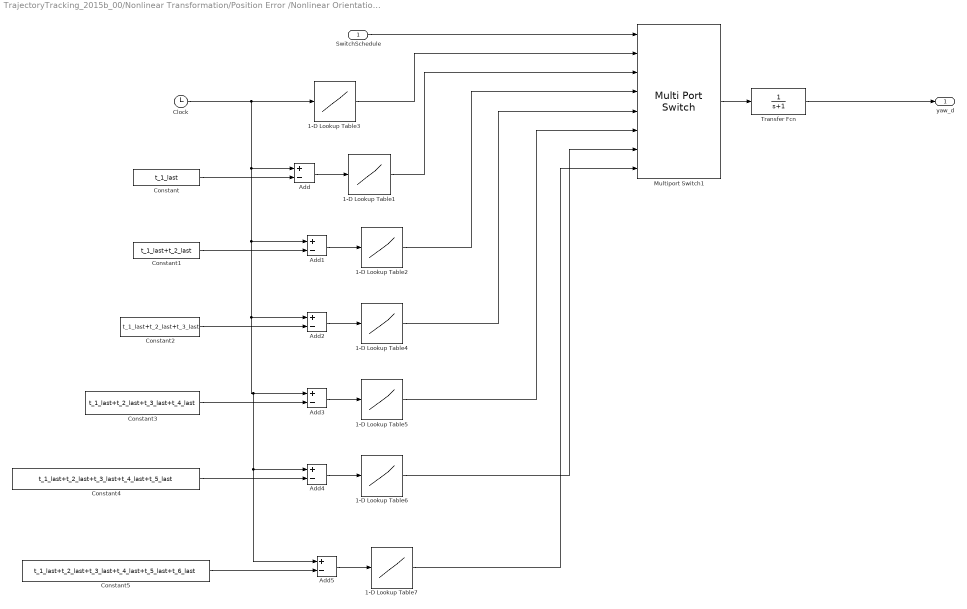
== system TrajectoryTracking_2015b_00/Nonlinear Transformation/Position Error /Nonlinear Orientation Transformation/yaw_error/theta_d ==
  SwitchSchedule : Inport
  1-D Lookup Table1 : Lookup_n-D  NumberOfTableDimensions=1  BreakpointsForDimension1=t_e_2  Table=yaw_angle_2  InternalRulePriority=Speed  RndMeth=Simplest  InputSameDT=on
  1-D Lookup Table2 : Lookup_n-D  NumberOfTableDimensions=1  BreakpointsForDimension1=t_e_3  Table=yaw_angle_3  InternalRulePriority=Speed  RndMeth=Simplest  InputSameDT=on
  1-D Lookup Table3 : Lookup_n-D  NumberOfTableDimensions=1  BreakpointsForDimension1=t_e_1  Table=yaw_angle_1  InternalRulePriority=Speed  RndMeth=Simplest  InputSameDT=on
  1-D Lookup Table4 : Lookup_n-D  NumberOfTableDimensions=1  BreakpointsForDimension1=t_e_4  Table=yaw_angle_4  InternalRulePriority=Speed  RndMeth=Simplest  InputSameDT=on
  1-D Lookup Table5 : Lookup_n-D  NumberOfTableDimensions=1  BreakpointsForDimension1=t_e_5  Table=yaw_angle_5  InternalRulePriority=Speed  RndMeth=Simplest  InputSameDT=on
  1-D Lookup Table6 : Lookup_n-D  NumberOfTableDimensions=1  BreakpointsForDimension1=t_e_6  Table=yaw_angle_6  InternalRulePriority=Speed  RndMeth=Simplest  InputSameDT=on
  1-D Lookup Table7 : Lookup_n-D  NumberOfTableDimensions=1  BreakpointsForDimension1=t_e_7  Table=yaw_angle_7  InternalRulePriority=Speed  RndMeth=Simplest  InputSameDT=on
  Add{,1..5} (6 alike) : Sum  Inputs=+-
  Clock : Clock
  Constant : Constant  Value=t_1_last
  Constant1 : Constant  Value=t_1_last+t_2_last
  Constant2 : Constant  Value=t_1_last+t_2_last+t_3_last
  Constant3 : Constant  Value=t_1_last+t_2_last+t_3_last+t_4_last
  Constant4 : Constant  Value=t_1_last+t_2_last+t_3_last+t_4_last+t_5_last
  Constant5 : Constant  Value=t_1_last+t_2_last+t_3_last+t_4_last+t_5_last+t_6_last
  Multiport Switch1 : MultiPortSwitch  Inputs=7
  Transfer Fcn : TransferFcn  Denominator=[1 1]
  yaw_d : Outport
  wires:
  SwitchSchedule/1 -> Multiport Switch1/1
  1-D Lookup Table1/1 -> Multiport Switch1/3
  1-D Lookup Table3/1 -> Multiport Switch1/2
  Constant/1 -> Add/2
  Multiport Switch1/1 -> Transfer Fcn/1
  Clock/1 -> Add5/1, Add4/1, Add3/1, Add2/1, Add1/1, Add/1, 1-D Lookup Table3/1
  Add/1 -> 1-D Lookup Table1/1
  Add1/1 -> 1-D Lookup Table2/1
  Constant1/1 -> Add1/2
  1-D Lookup Table2/1 -> Multiport Switch1/4
  Constant2/1 -> Add2/2
  Add2/1 -> 1-D Lookup Table4/1
  1-D Lookup Table4/1 -> Multiport Switch1/5
  Add3/1 -> 1-D Lookup Table5/1
  Constant3/1 -> Add3/2
  1-D Lookup Table5/1 -> Multiport Switch1/6
  Add4/1 -> 1-D Lookup Table6/1
  Constant4/1 -> Add4/2
  1-D Lookup Table6/1 -> Multiport Switch1/7
  Add5/1 -> 1-D Lookup Table7/1
  Constant5/1 -> Add5/2
  1-D Lookup Table7/1 -> Multiport Switch1/8
  Transfer Fcn/1 -> yaw_d/1

== system TrajectoryTracking_2015b_00/Nonlinear Transformation/Position Error /Nonlinear Position Transformation/x_error/x_d ==
  SwitchSchedule : Inport
  1-D Lookup Table1 : Lookup_n-D  NumberOfTableDimensions=1  BreakpointsForDimension1=t_e_3  Table=x3  InternalRulePriority=Speed  RndMeth=Simplest  InputSameDT=on
  1-D Lookup Table2 : Lookup_n-D  NumberOfTableDimensions=1  BreakpointsForDimension1=t_e_4  Table=x4  InternalRulePriority=Speed  RndMeth=Simplest  InputSameDT=on
  1-D Lookup Table3 : Lookup_n-D  NumberOfTableDimensions=1  BreakpointsForDimension1=t_e_5  Table=x5  InternalRulePriority=Speed  RndMeth=Simplest  InputSameDT=on
  1-D Lookup Table4 : Lookup_n-D  NumberOfTableDimensions=1  BreakpointsForDimension1=t_e_6  Table=x6  InternalRulePriority=Speed  RndMeth=Simplest  InputSameDT=on
  1-D Lookup Table5 : Lookup_n-D  NumberOfTableDimensions=1  BreakpointsForDimension1=t_e_7  Table=x7  InternalRulePriority=Speed  RndMeth=Simplest  InputSameDT=on
  1-D Lookup Table7 : Lookup_n-D  NumberOfTableDimensions=1  BreakpointsForDimension1=t_e_2  Table=x2  InternalRulePriority=Speed  RndMeth=Simplest  InputSameDT=on
  1-D Lookup Table9 : Lookup_n-D  NumberOfTableDimensions=1  BreakpointsForDimension1=t_e_1  Table=x1  InternalRulePriority=Speed  RndMeth=Simplest  InputSameDT=on
  Add{,1..5} (6 alike) : Sum  Inputs=+-
  Clock : Clock
  Constant : Constant  Value=t_1_last
  Constant1 : Constant  Value=t_1_last+t_2_last
  Constant2 : Constant  Value=t_1_last+t_2_last+t_3_last
  Constant3 : Constant  Value=t_1_last+t_2_last+t_3_last+t_4_last
  Constant4 : Constant  Value=t_1_last+t_2_last+t_3_last+t_4_last+t_5_last
  Constant5 : Constant  Value=t_1_last+t_2_last+t_3_last+t_4_last+t_5_last+t_6_last
  Multiport Switch1 : MultiPortSwitch  Inputs=7
  Transfer Fcn1 : TransferFcn  Denominator=[1 1]
  x_d : Outport
  wires:
  1-D Lookup Table7/1 -> Multiport Switch1/3
  1-D Lookup Table9/1 -> Multiport Switch1/2
  Constant/1 -> Add/2
  Multiport Switch1/1 -> Transfer Fcn1/1
  SwitchSchedule/1 -> Multiport Switch1/1
  Add/1 -> 1-D Lookup Table7/1
  Constant1/1 -> Add1/2
  Add1/1 -> 1-D Lookup Table1/1
  1-D Lookup Table1/1 -> Multiport Switch1/4
  Add2/1 -> 1-D Lookup Table2/1
  Constant2/1 -> Add2/2
  1-D Lookup Table2/1 -> Multiport Switch1/5
  Transfer Fcn1/1 -> x_d/1
  Clock/1 -> Add1/1, Add5/1, Add4/1, Add3/1, Add2/1, Add/1, 1-D Lookup Table9/1
  Constant3/1 -> Add3/2
  Add3/1 -> 1-D Lookup Table3/1
  1-D Lookup Table3/1 -> Multiport Switch1/6
  Add4/1 -> 1-D Lookup Table4/1
  Constant4/1 -> Add4/2
  1-D Lookup Table4/1 -> Multiport Switch1/7
  Add5/1 -> 1-D Lookup Table5/1
  Constant5/1 -> Add5/2
  1-D Lookup Table5/1 -> Multiport Switch1/8

== system TrajectoryTracking_2015b_00/Nonlinear Transformation/Position Error /Nonlinear Position Transformation/y_error/y_d ==
  SwitchSchedule : Inport
  1-D Lookup Table1 : Lookup_n-D  NumberOfTableDimensions=1  BreakpointsForDimension1=t_e_3  Table=y3  InternalRulePriority=Speed  RndMeth=Simplest  InputSameDT=on
  1-D Lookup Table10 : Lookup_n-D  NumberOfTableDimensions=1  BreakpointsForDimension1=t_e_1  Table=y1  InternalRulePriority=Speed  RndMeth=Simplest  InputSameDT=on
  1-D Lookup Table2 : Lookup_n-D  NumberOfTableDimensions=1  BreakpointsForDimension1=t_e_4  Table=y4  InternalRulePriority=Speed  RndMeth=Simplest  InputSameDT=on
  1-D Lookup Table3 : Lookup_n-D  NumberOfTableDimensions=1  BreakpointsForDimension1=t_e_5  Table=y5  InternalRulePriority=Speed  RndMeth=Simplest  InputSameDT=on
  1-D Lookup Table4 : Lookup_n-D  NumberOfTableDimensions=1  BreakpointsForDimension1=t_e_7  Table=y7  InternalRulePriority=Speed  RndMeth=Simplest  InputSameDT=on
  1-D Lookup Table5 : Lookup_n-D  NumberOfTableDimensions=1  BreakpointsForDimension1=t_e_6  Table=y6  InternalRulePriority=Speed  RndMeth=Simplest  InputSameDT=on
  1-D Lookup Table8 : Lookup_n-D  NumberOfTableDimensions=1  BreakpointsForDimension1=t_e_2  Table=y2  InternalRulePriority=Speed  RndMeth=Simplest  InputSameDT=on
  Add{,1..5} (6 alike) : Sum  Inputs=+-
  Clock : Clock
  Constant : Constant  Value=t_1_last
  Constant1 : Constant  Value=t_1_last+t_2_last
  Constant2 : Constant  Value=t_1_last+t_2_last+t_3_last
  Constant3 : Constant  Value=t_1_last+t_2_last+t_3_last+t_4_last
  Constant4 : Constant  Value=t_1_last+t_2_last+t_3_last+t_4_last+t_5_last
  Constant5 : Constant  Value=t_1_last+t_2_last+t_3_last+t_4_last+t_5_last+t_6_last
  Multiport Switch : MultiPortSwitch  Inputs=7
  Transfer Fcn : TransferFcn  Denominator=[1 1]
  y_d : Outport
  wires:
  1-D Lookup Table8/1 -> Multiport Switch/3
  1-D Lookup Table10/1 -> Multiport Switch/2
  Constant/1 -> Add/2
  Multiport Switch/1 -> Transfer Fcn/1
  Add/1 -> 1-D Lookup Table8/1
  SwitchSchedule/1 -> Multiport Switch/1
  Constant1/1 -> Add1/2
  1-D Lookup Table1/1 -> Multiport Switch/4
  Add1/1 -> 1-D Lookup Table1/1
  Clock/1 -> Add4/1, Add5/1, Add3/1, Add2/1, Add1/1, Add/1, 1-D Lookup Table10/1
  Add2/1 -> 1-D Lookup Table2/1
  Constant2/1 -> Add2/2
  1-D Lookup Table2/1 -> Multiport Switch/5
  Transfer Fcn/1 -> y_d/1
  Constant3/1 -> Add3/2
  Add3/1 -> 1-D Lookup Table3/1
  1-D Lookup Table3/1 -> Multiport Switch/6
  Constant5/1 -> Add4/2
  Add4/1 -> 1-D Lookup Table4/1
  Constant4/1 -> Add5/2
  Add5/1 -> 1-D Lookup Table5/1
  1-D Lookup Table5/1 -> Multiport Switch/7
  1-D Lookup Table4/1 -> Multiport Switch/8

== system TrajectoryTracking_2015b_00/Nonlinear Transformation/Position Error /Nonlinear Position Transformation/z_error/z_d ==
  SwitchSchedule : Inport
  1-D Lookup Table1 : Lookup_n-D  NumberOfTableDimensions=1  BreakpointsForDimension1=t_e_2  Table=z2  InternalRulePriority=Speed  RndMeth=Simplest  InputSameDT=on
  1-D Lookup Table2 : Lookup_n-D  NumberOfTableDimensions=1  BreakpointsForDimension1=t_e_3  Table=z3  InternalRulePriority=Speed  RndMeth=Simplest  InputSameDT=on
  1-D Lookup Table3 : Lookup_n-D  NumberOfTableDimensions=1  BreakpointsForDimension1=t_e_1  Table=z1  InternalRulePriority=Speed  RndMeth=Simplest  InputSameDT=on
  1-D Lookup Table4 : Lookup_n-D  NumberOfTableDimensions=1  BreakpointsForDimension1=t_e_4  Table=z4  InternalRulePriority=Speed  RndMeth=Simplest  InputSameDT=on
  1-D Lookup Table5 : Lookup_n-D  NumberOfTableDimensions=1  BreakpointsForDimension1=t_e_5  Table=z5  InternalRulePriority=Speed  RndMeth=Simplest  InputSameDT=on
  1-D Lookup Table6 : Lookup_n-D  NumberOfTableDimensions=1  BreakpointsForDimension1=t_e_6  Table=z6  InternalRulePriority=Speed  RndMeth=Simplest  InputSameDT=on
  1-D Lookup Table7 : Lookup_n-D  NumberOfTableDimensions=1  BreakpointsForDimension1=t_e_7  Table=z7  InternalRulePriority=Speed  RndMeth=Simplest  InputSameDT=on
  Add{,1..5} (6 alike) : Sum  Inputs=+-
  Clock : Clock
  Constant1 : Constant  Value=t_1_last+t_2_last+t_3_last+t_4_last
  Constant2 : Constant  Value=t_1_last
  Constant3 : Constant  Value=t_1_last+t_2_last
  Constant4 : Constant  Value=t_1_last+t_2_last+t_3_last
  Constant5 : Constant  Value=t_1_last+t_2_last+t_3_last+t_4_last+t_5_last
  Constant6 : Constant  Value=t_1_last+t_2_last+t_3_last+t_4_last+t_5_last+t_6_last
  Multiport Switch : MultiPortSwitch  Inputs=7
  Transfer Fcn : TransferFcn  Denominator=[1 1]
  z_d : Outport
  wires:
  1-D Lookup Table1/1 -> Multiport Switch/3
  1-D Lookup Table3/1 -> Multiport Switch/2
  Constant2/1 -> Add/2
  Multiport Switch/1 -> Transfer Fcn/1
  Add/1 -> 1-D Lookup Table1/1
  SwitchSchedule/1 -> Multiport Switch/1
  1-D Lookup Table2/1 -> Multiport Switch/4
  Add1/1 -> 1-D Lookup Table2/1
  Constant3/1 -> Add1/2
  Add2/1 -> 1-D Lookup Table4/1
  Clock/1 -> Add5/1, Add4/1, Add3/1, Add2/1, Add1/1, Add/1, 1-D Lookup Table3/1
  1-D Lookup Table4/1 -> Multiport Switch/5
  Constant4/1 -> Add2/2
  Transfer Fcn/1 -> z_d/1
  Add3/1 -> 1-D Lookup Table5/1
  Constant1/1 -> Add3/2
  1-D Lookup Table5/1 -> Multiport Switch/6
  Add4/1 -> 1-D Lookup Table6/1
  Constant5/1 -> Add4/2
  1-D Lookup Table6/1 -> Multiport Switch/7
  Constant6/1 -> Add5/2
  Add5/1 -> 1-D Lookup Table7/1
  1-D Lookup Table7/1 -> Multiport Switch/8

== system TrajectoryTracking_2015b_00/Underwater Robot System/Underwater Robot System/Underwater Robot Dynamics /6DOF Coriolis forces/3x3 cross product ==
  a : Inport
  b : Inport  Port=2
  Product : Product  SaturateOnIntegerOverflow=on  InputSameDT=on  OutDataTypeStr=Inherit: Same as first input
  Product1 : Product  SaturateOnIntegerOverflow=on  InputSameDT=on  OutDataTypeStr=Inherit: Same as first input
  Selector : Selector  InputPortWidth=3  IndexOptions=Index vector (dialog)  Indices=[2 3 1]  OutputSizes=1
  Selector1 : Selector  InputPortWidth=3  IndexOptions=Index vector (dialog)  Indices=[3 1 2]  OutputSizes=1
  Selector2 : Selector  InputPortWidth=3  IndexOptions=Index vector (dialog)  Indices=[2 3 1]  OutputSizes=1
  Selector3 : Selector  InputPortWidth=3  IndexOptions=Index vector (dialog)  Indices=[3 1 2]  OutputSizes=1
  Sum : Sum  Inputs=+|-  SaturateOnIntegerOverflow=on  InputSameDT=on  OutDataTypeStr=Inherit: Same as first input
  c : Outport  InitialOutput=0
  wires:
  Selector3/1 -> Product1/1
  Selector2/1 -> Product1/2
  Product1/1 -> Sum/2
  Selector1/1 -> Product/2
  Product/1 -> Sum/1
  a/1 -> Selector3/1, Selector/1
  Selector/1 -> Product/1
  b/1 -> Selector2/1, Selector1/1
  Sum/1 -> c/1

== system TrajectoryTracking_2015b_00/Underwater Robot System/Underwater Robot System/Underwater Robot Dynamics /6DOF Coriolis forces/3x3 cross product 1 ==
  a : Inport
  b : Inport  Port=2
  Product : Product  SaturateOnIntegerOverflow=on  InputSameDT=on  OutDataTypeStr=Inherit: Same as first input
  Product1 : Product  SaturateOnIntegerOverflow=on  InputSameDT=on  OutDataTypeStr=Inherit: Same as first input
  Selector : Selector  InputPortWidth=3  IndexOptions=Index vector (dialog)  Indices=[2 3 1]  OutputSizes=1
  Selector1 : Selector  InputPortWidth=3  IndexOptions=Index vector (dialog)  Indices=[3 1 2]  OutputSizes=1
  Selector2 : Selector  InputPortWidth=3  IndexOptions=Index vector (dialog)  Indices=[2 3 1]  OutputSizes=1
  Selector3 : Selector  InputPortWidth=3  IndexOptions=Index vector (dialog)  Indices=[3 1 2]  OutputSizes=1
  Sum : Sum  Inputs=+|-  SaturateOnIntegerOverflow=on  InputSameDT=on  OutDataTypeStr=Inherit: Same as first input
  c : Outport  InitialOutput=0
  wires:
  Selector3/1 -> Product1/1
  Selector2/1 -> Product1/2
  Product1/1 -> Sum/2
  Selector1/1 -> Product/2
  Product/1 -> Sum/1
  a/1 -> Selector3/1, Selector/1
  Selector/1 -> Product/1
  b/1 -> Selector2/1, Selector1/1
  Sum/1 -> c/1

== system TrajectoryTracking_2015b_00/Underwater Robot System/Underwater Robot System/Underwater Robot Dynamics /6DOF Coriolis forces/3x3 cross product 2 ==
  a : Inport
  b : Inport  Port=2
  Product : Product  SaturateOnIntegerOverflow=on  InputSameDT=on  OutDataTypeStr=Inherit: Same as first input
  Product1 : Product  SaturateOnIntegerOverflow=on  InputSameDT=on  OutDataTypeStr=Inherit: Same as first input
  Selector : Selector  InputPortWidth=3  IndexOptions=Index vector (dialog)  Indices=[2 3 1]  OutputSizes=1
  Selector1 : Selector  InputPortWidth=3  IndexOptions=Index vector (dialog)  Indices=[3 1 2]  OutputSizes=1
  Selector2 : Selector  InputPortWidth=3  IndexOptions=Index vector (dialog)  Indices=[2 3 1]  OutputSizes=1
  Selector3 : Selector  InputPortWidth=3  IndexOptions=Index vector (dialog)  Indices=[3 1 2]  OutputSizes=1
  Sum : Sum  Inputs=+|-  SaturateOnIntegerOverflow=on  InputSameDT=on  OutDataTypeStr=Inherit: Same as first input
  c : Outport  InitialOutput=0
  wires:
  Selector3/1 -> Product1/1
  Selector2/1 -> Product1/2
  Product1/1 -> Sum/2
  Selector1/1 -> Product/2
  Product/1 -> Sum/1
  a/1 -> Selector3/1, Selector/1
  Selector/1 -> Product/1
  b/1 -> Selector2/1, Selector1/1
  Sum/1 -> c/1

== matlab function TrajectoryTracking_2015b_00/Switch Control ==
  data: u input; y output
function y = SwitchSchedule(u)
%% in this function 
if(u>=40 && u<=60)
    y=2;
elseif(u>60 && u<=80)
    y=3;
elseif(u>80 && u<=120)
    y=4;
elseif(u>120 && u<=140)
    y=5;
elseif(u>140 && u<=160)
    y=6;
elseif(u>160 && u<=200)
    y=7;
else
    y=1;
end
